simulink model "ITireAppMdlSiL"  (R2017b)
settings: Solver=FixedStepAuto  StartTime=0.0  StopTime=10000  FixedStep=0.1  RelTol=1e-3
model workspace (MAT data in the model file):
  AilrflowValidFlag1 = [0.01235 0.03834 0.06233 0.08839 0.11261 0.13833 0.16348 0.18843 0.2134 0.23767 0.26241 0.28847 ... (108920 elements, 54460x2)]
  AilrflowValidFlag2 = [0.01258 0.03858 0.06256 0.08863 0.11285 0.13856 0.16371 0.18866 0.21363 0.2379 0.26264 0.2887 ... (108920 elements, 54460x2)]
  Airflow = [0.01258 0.03858 0.06256 0.08863 0.11285 0.13856 0.16371 0.18866 0.21363 0.2379 0.26264 0.2887 ... (108920 elements, 54460x2)]
  Frequency = [0.01235 0.03834 0.06233 0.08839 0.11261 0.13833 0.16348 0.18843 0.2134 0.23767 0.26241 0.28847 ... (108920 elements, 54460x2)]
  IntkAirHmdty = [0.07576 0.17591 0.27589 0.37591 0.47621 0.5753 0.67605 0.77531 0.87537 0.97532 1.07528 1.17533 ... (27230 elements, 13615x2)]
  IntkAirTemp = [0.07576 0.17591 0.27589 0.37591 0.47621 0.5753 0.67605 0.77531 0.87537 0.97532 1.07528 1.17533 ... (27230 elements, 13615x2)]
  IntkHmdtyTemp = [0.07576 0.17591 0.27589 0.37591 0.47621 0.5753 0.67605 0.77531 0.87537 0.97532 1.07528 1.17533 ... (27230 elements, 13615x2)]
  PriPresFilterValue = [0.01235 0.03834 0.06233 0.08839 0.11261 0.13833 0.16348 0.18843 0.2134 0.23767 0.26241 0.28847 ... (108920 elements, 54460x2)]
  PriPresRawValue = [0.01235 0.03834 0.06233 0.08839 0.11261 0.13833 0.16348 0.18843 0.2134 0.23767 0.26241 0.28847 ... (108920 elements, 54460x2)]
  SecPresFilterValue = [0.01258 0.03858 0.06256 0.08863 0.11285 0.13856 0.16371 0.18866 0.21363 0.2379 0.26264 0.2887 ... (108920 elements, 54460x2)]
  SecPresRawValue = [0.01258 0.03858 0.06256 0.08863 0.11285 0.13856 0.16371 0.18866 0.21363 0.2379 0.26264 0.2887 ... (108920 elements, 54460x2)]
  deltaPriPresFilterV = [0.01235 0.03834 0.06233 0.08839 0.11261 0.13833 0.16348 0.18843 0.2134 0.23767 0.26241 0.28847 ... (108920 elements, 54460x2)]
  deltaPriPresRawValu = [0.01235 0.03834 0.06233 0.08839 0.11261 0.13833 0.16348 0.18843 0.2134 0.23767 0.26241 0.28847 ... (108920 elements, 54460x2)]
  deltaSecPresFilterV = [0.01258 0.03858 0.06256 0.08863 0.11285 0.13856 0.16371 0.18866 0.21363 0.2379 0.26264 0.2887 ... (108920 elements, 54460x2)]
  deltaSecPresRawValu = [0.01258 0.03858 0.06256 0.08863 0.11285 0.13856 0.16371 0.18866 0.21363 0.2379 0.26264 0.2887 ... (108920 elements, 54460x2)]
undefined symbols (not defined in the file or in its folder): sigbuilder_block
(part 1 of 2)
settings Model: DataDictionary=ITiremyDictionary.sldd  Creator=xiangyinl  LastModifiedBy=Bigcat
settings DataIOCC: SaveOutput=off
settings OptimizationCC: DefaultParameterBehavior=Inlined  UseDivisionForNetSlopeComputation=on  UseSpecifiedMinMax=on  InlineInvariantSignals=on  EnhancedBackFolding=on  PassReuseOutputArgsAs=Individual arguments  ZeroExternalMemoryAtStartup=off  InitFltsAndDblsToZero=on  LifeSpan=inf  DifferentSizesBufferReuse=on
settings DebuggingCC: SignalInfNanChecking=error  ReadBeforeWriteMsg=EnableAllAsError  WriteAfterWriteMsg=EnableAllAsError  WriteAfterReadMsg=EnableAllAsError  IntegerOverflowMsg=error  ParameterTunabilityLossMsg=error  UniqueDataStoreMsg=error  AssertControl=DisableAll  StrictBusMsg=ErrorOnBusTreatedAsVector  NonBusSignalsTreatedAsBus=error  SFInvalidInputDataAccessInChartInitDiag=error  SFTransitionOutsideNaturalParentDiag=error  SFUnreachableExecutionPathDiag=error  SFUndirectedBroadcastEventsDiag=error  SFOutputUsedAsStateInMooreChartDiag=none  IntegerSaturationMsg=error
settings HardwareCC: ProdBitPerPointer=32  ProdBitPerSizeT=32  ProdBitPerPtrDiffT=32  ProdLargestAtomicInteger=Integer  ProdWordSize=32  ProdHWDeviceType=STMicroelectronics->STM32 32-bit Cortex-M
settings ModelReferenceCC: ModelReferenceNumInstancesAllowed=Single
settings SFSimCC: MATLABDynamicMemAlloc=off
settings RTWCC: SystemTargetFile=ert.tlc  TemplateMakefile=ert_default_tmf  GenerateReport=on  Toolchain=Microsoft Visual C++ 2015 v14.0 | nmake (64-bit Windows)  IncludeHyperlinkInReport=on  LaunchReport=on  GenerateTraceInfo=on  GenerateTraceReport=on  GenerateTraceReportSl=on  GenerateTraceReportSf=on  GenerateTraceReportEml=on
settings CodeAppCC: ForceParamTrailComments=on  IgnoreCustomStorageClasses=off  OperatorAnnotations=on  SimulinkDataObjDesc=on  SFDataObjDesc=on  MATLABFcnDesc=on  InsertBlockDesc=on  StateflowObjectComments=on  MATLABSourceComments=on  EnableCustomComments=on  ReqsInCode=on
settings ERTTargetCC: TargetLangStandard=C99 (ISO)  GenerateSampleERTMain=on  CombineSignalStateStructs=on  SuppressErrorStatus=on  SupportNonFinite=off  ParenthesesLevel=Maximum  CastingMode=Standards  GenerateSharedConstants=off  ERTCustomFileTemplate=example_file_process.tlc  ERTFilePackagingFormat=Compact  ConvertIfToSwitch=off  EnableSignedLeftShifts=off  EnableSignedRightShifts=off

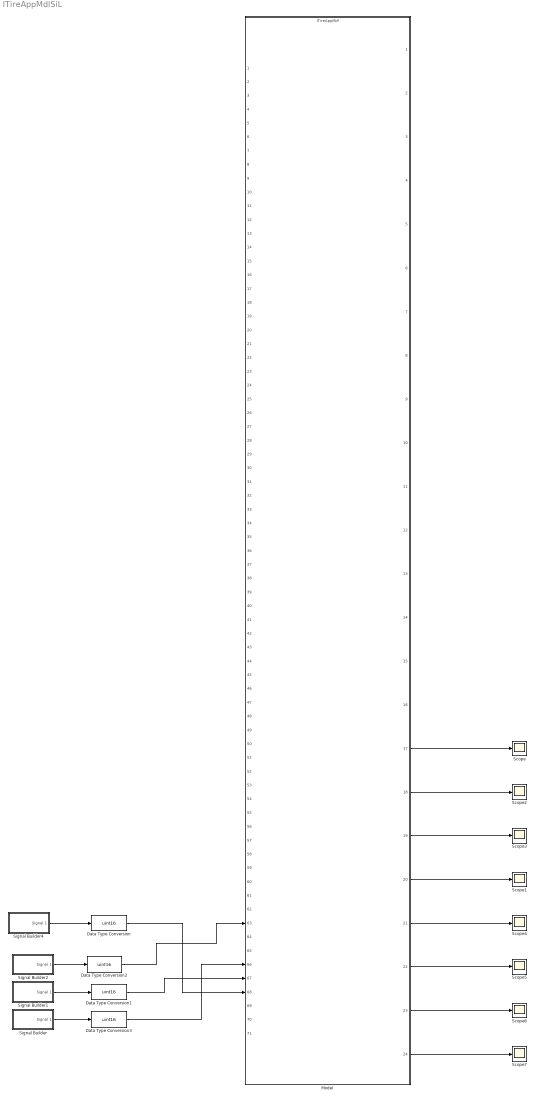
== system ITireAppMdlSiL ==
  Data Type Conversion{,1..3} (4 alike) : DataTypeConversion  OutDataTypeStr=uint16
  Model : ModelReference  ModelNameDialog=ITireAppMdl.slx  SimulationMode=Normal  ShowModelTerminatePort=on  ModelReferenceVersion=1.126
  Scope{,1..7} (8 alike) : Scope
  Signal Builder : Subsystem  Tag=STV Subsys  LoadFcn=sigbuilder_block('load');  StartFcn=sigbuilder_block('start');  StopFcn=sigbuilder_block('stop');  ClipboardFcn=sigbuilder_block('clipboard');  mask(Sigbuilder block){tuvar=[0:10]}
      mask help: Simulink:masks:SigbuilderBlock_MD
      mask init:
      | if ~strcmp(get_param(bdroot(gcbh),'SimulationStatus'),'stopped') tuvar = sigbuilder_block('maskInit'); end
      settings: CopyFcn=sigbuilder_block('copy');  DeleteFcn=sigbuilder_block('delete');  ModelCloseFcn=sigbuilder_block('modelClose');  PreSaveFcn=sigbuilder_block('preSave');  PauseFcn=sigbuilder_block('pause');  ContinueFcn=sigbuilder_block('continue');  NameChangeFcn=sigbuilder_block('namechange');  OpenFcn=sigbuilder_block('open',[437.4 186.6 687.6 400.2 ]);  CloseFcn=sigbuilder_block('close');
      mask Display: plot(0, 0, 100, 100,[2, 2, 32, 32, 2], [68, 8, 8, 68, 68],[32, 2], [38, 38], [32, 19, 2],[53, 60, 44], [32, 17, 17, 2],[16, 16, 31, 31]);txt = getActiveGroup(gcbh);text(2, 100, txt,'verticalAlignment', 'top');
  Signal Builder1 : Subsystem  Tag=STV Subsys  LoadFcn=sigbuilder_block('load');  StartFcn=sigbuilder_block('start');  StopFcn=sigbuilder_block('stop');  ClipboardFcn=sigbuilder_block('clipboard');  mask(Sigbuilder block){tuvar=[0:10]}
      mask help: Simulink:masks:SigbuilderBlock_MD
      mask init:
      | if ~strcmp(get_param(bdroot(gcbh),'SimulationStatus'),'stopped') tuvar = sigbuilder_block('maskInit'); end
      settings: CopyFcn=sigbuilder_block('copy');  DeleteFcn=sigbuilder_block('delete');  ModelCloseFcn=sigbuilder_block('modelClose');  PreSaveFcn=sigbuilder_block('preSave');  PauseFcn=sigbuilder_block('pause');  ContinueFcn=sigbuilder_block('continue');  NameChangeFcn=sigbuilder_block('namechange');  OpenFcn=sigbuilder_block('open',[437.4 186.6 687.6 400.2 ]);  CloseFcn=sigbuilder_block('close');
      mask Display: plot(0, 0, 100, 100,[2, 2, 32, 32, 2], [68, 8, 8, 68, 68],[32, 2], [38, 38], [32, 19, 2],[53, 60, 44], [32, 17, 17, 2],[16, 16, 31, 31]);txt = getActiveGroup(gcbh);text(2, 100, txt,'verticalAlignment', 'top');
  Signal Builder2 : Subsystem  Tag=STV Subsys  LoadFcn=sigbuilder_block('load');  StartFcn=sigbuilder_block('start');  StopFcn=sigbuilder_block('stop');  ClipboardFcn=sigbuilder_block('clipboard');  mask(Sigbuilder block){tuvar=[0:10]}
      mask help: Simulink:masks:SigbuilderBlock_MD
      mask init:
      | if ~strcmp(get_param(bdroot(gcbh),'SimulationStatus'),'stopped') tuvar = sigbuilder_block('maskInit'); end
      settings: CopyFcn=sigbuilder_block('copy');  DeleteFcn=sigbuilder_block('delete');  ModelCloseFcn=sigbuilder_block('modelClose');  PreSaveFcn=sigbuilder_block('preSave');  PauseFcn=sigbuilder_block('pause');  ContinueFcn=sigbuilder_block('continue');  NameChangeFcn=sigbuilder_block('namechange');  OpenFcn=sigbuilder_block('open',[437.4 186.6 687.6 400.2 ]);  CloseFcn=sigbuilder_block('close');
      mask Display: plot(0, 0, 100, 100,[2, 2, 32, 32, 2], [68, 8, 8, 68, 68],[32, 2], [38, 38], [32, 19, 2],[53, 60, 44], [32, 17, 17, 2],[16, 16, 31, 31]);txt = getActiveGroup(gcbh);text(2, 100, txt,'verticalAlignment', 'top');
  Signal Builder4 : Subsystem  Tag=STV Subsys  LoadFcn=sigbuilder_block('load');  StartFcn=sigbuilder_block('start');  StopFcn=sigbuilder_block('stop');  ClipboardFcn=sigbuilder_block('clipboard');  mask(Sigbuilder block){tuvar=[0:10]}
      mask help: Simulink:masks:SigbuilderBlock_MD
      mask init:
      | if ~strcmp(get_param(bdroot(gcbh),'SimulationStatus'),'stopped') tuvar = sigbuilder_block('maskInit'); end
      settings: CopyFcn=sigbuilder_block('copy');  DeleteFcn=sigbuilder_block('delete');  ModelCloseFcn=sigbuilder_block('modelClose');  PreSaveFcn=sigbuilder_block('preSave');  PauseFcn=sigbuilder_block('pause');  ContinueFcn=sigbuilder_block('continue');  NameChangeFcn=sigbuilder_block('namechange');  OpenFcn=sigbuilder_block('open',[437.4 186.6 687.6 400.2 ]);  CloseFcn=sigbuilder_block('close');
      mask Display: plot(0, 0, 100, 100,[2, 2, 32, 32, 2], [68, 8, 8, 68, 68],[32, 2], [38, 38], [32, 19, 2],[53, 60, 44], [32, 17, 17, 2],[16, 16, 31, 31]);txt = getActiveGroup(gcbh);text(2, 100, txt,'verticalAlignment', 'top');
  wires:
  Model/17 -> Scope/1
  Model/20 -> Scope1/1
  Model/19 -> Scope3/1
  Model/18 -> Scope2/1
  Signal Builder2/1(Signal 1) -> Data Type Conversion2/1
  Signal Builder1/1(Signal 1) -> Data Type Conversion1/1
  Signal Builder/1(Signal 1) -> Data Type Conversion3/1
  Signal Builder4/1(Signal 1) -> Data Type Conversion/1
  Model/21 -> Scope4/1
  Model/22 -> Scope5/1
  Model/23 -> Scope6/1
  Model/24 -> Scope7/1
  Data Type Conversion2/1 -> Model/63
  Data Type Conversion3/1 -> Model/66
  Data Type Conversion1/1 -> Model/67
  Data Type Conversion/1 -> Model/68
